simulink model "Simulate_position_motor_controllers"  (R2014b)
settings: Solver=ode23t  SolverMode=SingleTasking  StartTime=0.0  StopTime=simtime  RelTol=1e-3
values from neighbouring files (symbols this model uses):
  c0 = (s2 + s1 + s0)/(1 + r0)    [pbutest.m]    (also in workshop1.m)
  c0_ = (s2_ + s1_ + s0_)/(1 + r0)    [pbutest.m]    (also in workshop1.m)
  d0 = (r0*(s1 + s2) - s0)/(1 + r0)    [pbutest.m]    (also in workshop1.m)
  d0_ = (r0*(s1_ + s2_))/(1 + r0)    [pbutest.m]    (also in workshop1.m)
  d1 = s2    [pbutest.m]    (also in workshop1.m)
  d1_ = s2_    [pbutest.m]    (also in workshop1.m)
  F_c = 1.5e-3    (= 0.0015)    [continuous_design.m]    (also in workshop1.m)
  J1 = 0.0006    [continuous_design.m]    (also in workshop1.m)
  Kb = 10    [workshop1.m]
  motor = motor_pars    [continuous_design.m]    (also in workshop1.m)
  n = 5    [continuous_design.m]    (also in workshop1.m)
  r0 = 2*Zeta*omega3-b+omega1+omega2    [continuous_design.m]    (also in pbutest.m = (-b1^3*p1*p2*p3*p4-b0*b1^2*p1*p2*p3-b0*b1^2*p1*p2*p4-b0*b1^2; workshop1.m = (-b1^3*p1*p2*p3*p4-b0*b1^2*p1*p2*p3-b0*b1^2*p1*p2*p4-b0*b1^2)
  R_sim = Rd.num{1}    [pbutest.m]    (also in workshop1.m)
  S_sim = Sd.num{1}    [pbutest.m]    (also in workshop1.m)
  T_sim = Td.num{1}    [pbutest.m]    (also in workshop1.m)
  Ts = 2*pi/ws    [continuous_design.m]    (also in pbutest.m = 0.0108705628152; workshop1.m = 0.108705628152)
libraries: simulink x1
settings Model: Creator=Gabriel  LastModifiedBy=es2lab2
settings SolverCC: ZeroCrossAlgorithm=Adaptive
settings OptimizationCC: BlockReduction=off  BooleanDataType=off  UseDivisionForNetSlopeComputation=off  SimCompilerOptimization=off
settings DebuggingCC: SaveWithParameterizedLinksMsg=none  UnderspecifiedInitializationDetection=Classic  MergeDetectMultiDrivingBlocksExec=none  SignalResolutionControl=TryResolveAllWithWarning  SolverPrmCheckMsg=none  FrameProcessingCompatibilityMsg=error  AllowSymbolicDim=off
settings HardwareCC: TargetBitPerPointer=64  TargetLongLongMode=on  TargetIntDivRoundTo=Zero  TargetEndianess=LittleEndian  TargetWordSize=64  TargetHWDeviceType=MATLAB Host  ProdEqTarget=off
settings RTWCC: RTWCompilerOptimization=off
settings ConfigComp: CovMetricSettings=dw  CovHtmlReporting=on  CovSaveCumulativeToWorkspaceVar=on  CovSaveSingleToWorkspaceVar=on  CovModelRefEnable=Off  CovExternalEMLEnable=off  CovSFcnEnable=off

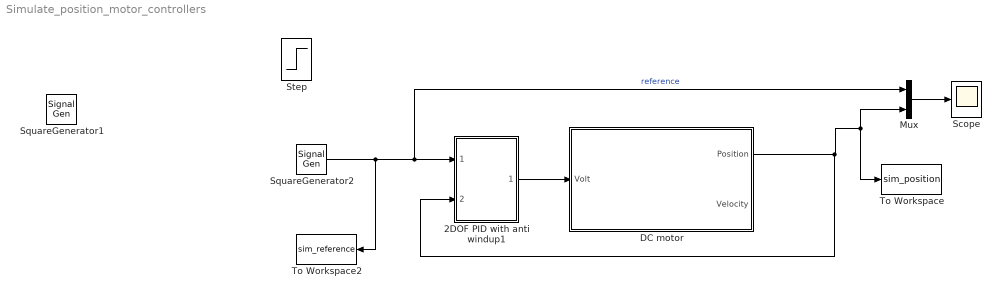
== system Simulate_position_motor_controllers ==
  2DOF PID with anti windup1 : Subsystem
  DC motor : Subsystem
  Mux : Mux  Inputs=2
  Scope : Scope
      settings: ShowLegends=on  TimeRange=7.551351351351352  YMin=-0.5  YMax=4.5
  SquareGenerator1 : SignalGenerator  WaveForm=square  Amplitude=4  Units=rad/sec
  SquareGenerator2 : SignalGenerator  WaveForm=square  Amplitude=4  Units=rad/sec
  Step : Step  Time=0  After=4  SampleTime=0
  To Workspace : ToWorkspace  VariableName=sim_position  SaveFormat=Timeseries  SampleTime=-1
  To Workspace2 : ToWorkspace  VariableName=sim_reference  SaveFormat=Timeseries  SampleTime=-1
  wires:
  SquareGenerator2/1 -> To Workspace2/1, Mux/1, 2DOF PID with anti windup1/1("reference ")  "reference"
  DC motor/1(Position) -> 2DOF PID with anti windup1/2(feedback), Mux/2, To Workspace/1
  2DOF PID with anti windup1/1(Voltage) -> DC motor/1(Volt)
  Mux/1 -> Scope/1

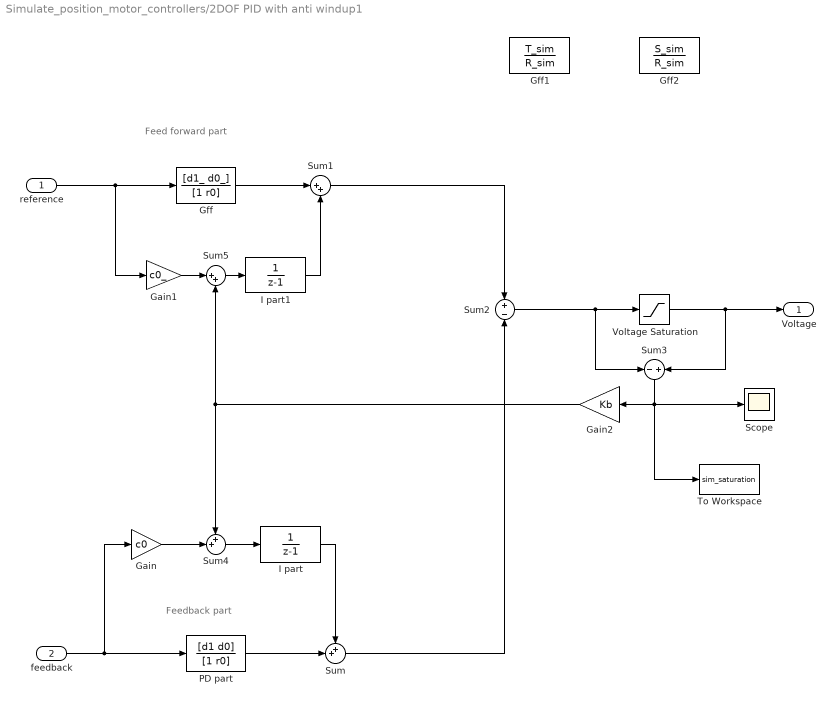
== system Simulate_position_motor_controllers/2DOF PID with anti windup1 ==
  note: Feedback part
  note: Feed forward part
  "reference " : Inport
  feedback : Inport  Port=2
  Gain : Gain  Gain=c0
  Gain1 : Gain  Gain=c0_
  Gain2 : Gain  Gain=Kb
  Gff : DiscreteTransferFcn  Numerator=[d1_ d0_]  Denominator=[1 r0]  SampleTime=Ts
  Gff1 : DiscreteTransferFcn  Numerator=T_sim  Denominator=R_sim  SampleTime=Ts
  Gff2 : DiscreteTransferFcn  Numerator=S_sim  Denominator=R_sim  SampleTime=Ts
  I part : DiscreteTransferFcn  Numerator=[0 1]  Denominator=[1 -1]  SampleTime=Ts
  I part1 : DiscreteTransferFcn  Numerator=[0 1]  Denominator=[1 -1]  SampleTime=Ts
  PD part : DiscreteTransferFcn  Numerator=[d1 d0]  Denominator=[1 r0]  SampleTime=Ts
  Scope : Scope
  Sum : Sum  Inputs=++|
  Sum1 : Sum  Inputs=|++
  Sum2 : Sum  Inputs=+|-
  Sum3 : Sum  Inputs=-|+
  Sum4 : Sum  Inputs=++|
  Sum5 : Sum  Inputs=|++
  To Workspace : ToWorkspace  VariableName=sim_saturation  SaveFormat=Timeseries  SampleTime=-1
  "Voltage Saturation " : Saturate  UpperLimit=24  LowerLimit=-24
  Voltage : Outport
  wires:
  "Voltage Saturation "/1 -> Sum3/2, Voltage/1
  "reference "/1 -> Gain1/1, Gff/1
  feedback/1 -> Gain/1, PD part/1
  Sum2/1 -> Sum3/1, "Voltage Saturation "/1
  Sum/1 -> Sum2/2
  Gff/1 -> Sum1/1
  I part1/1 -> Sum1/2
  Sum1/1 -> Sum2/1
  PD part/1 -> Sum/2
  I part/1 -> Sum/1
  Sum3/1 -> To Workspace/1, Scope/1, Gain2/1
  Sum4/1 -> I part/1
  Gain/1 -> Sum4/2
  Gain2/1 -> Sum5/2, Sum4/1
  Gain1/1 -> Sum5/1
  Sum5/1 -> I part1/1

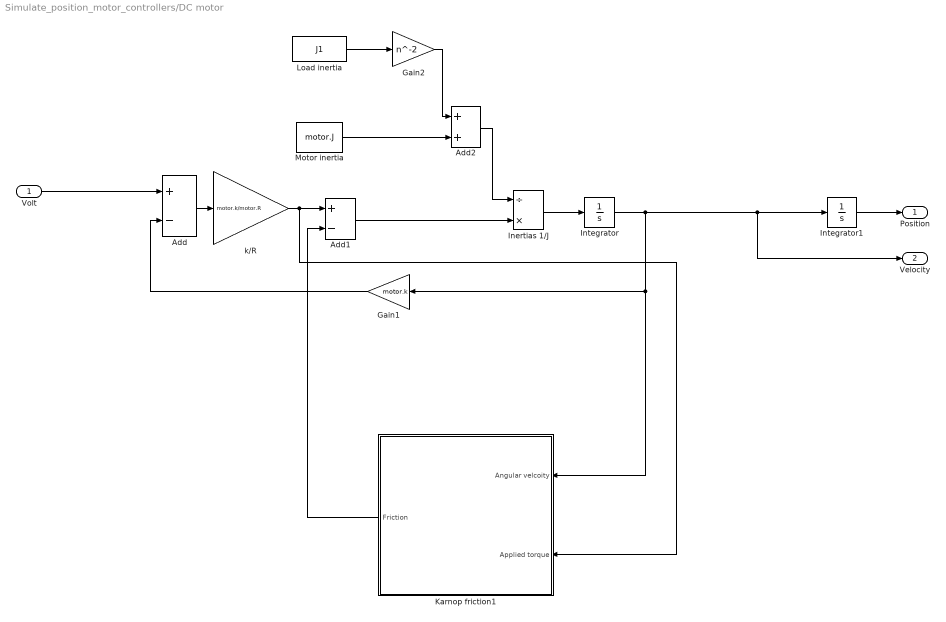
== system Simulate_position_motor_controllers/DC motor ==
  Volt : Inport
  Add : Sum  Inputs=+-
  Add1 : Sum  Inputs=+-
  Add2 : Sum
  Gain1 : Gain  Gain=motor.k
  Gain2 : Gain  Gain=n^-2
  Inertias 1/J : Product  Inputs=/*
  Integrator : Integrator
  Integrator1 : Integrator
  Karnop friction1 : Subsystem
  Load inertia : Constant  Value=J1
  Motor inertia : Constant  Value=motor.J
  "k/R " : Gain  Gain=motor.k/motor.R
  Position : Outport
  Velocity : Outport  Port=2
  wires:
  Karnop friction1/1(Friction) -> Add1/2
  Add2/1 -> Inertias 1/J/1
  Gain2/1 -> Add2/1
  Load inertia/1 -> Gain2/1
  Motor inertia/1 -> Add2/2
  Integrator/1 -> Integrator1/1, Velocity/1, Karnop friction1/1(Angular velcoity), Gain1/1
  Volt/1 -> Add/1
  Add1/1 -> Inertias 1/J/2
  Integrator1/1 -> Position/1
  Inertias 1/J/1 -> Integrator/1
  "k/R "/1 -> Add1/1, Karnop friction1/2(Applied torque)
  Add/1 -> "k/R "/1
  Gain1/1 -> Add/2

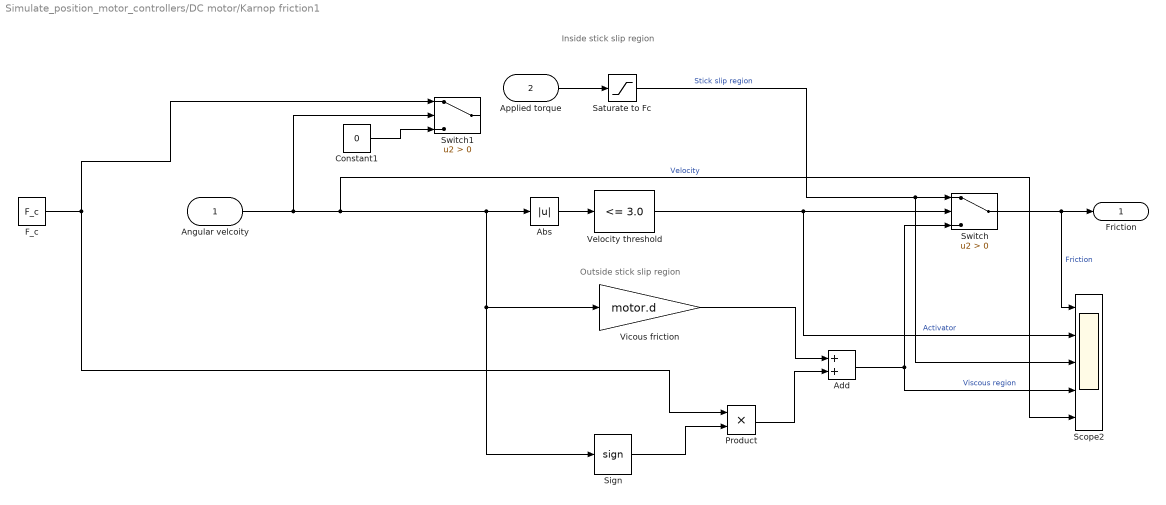
== system Simulate_position_motor_controllers/DC motor/Karnop friction1 ==
  note: Outside stick slip region
  note: Inside stick slip region
  Angular velcoity : Inport
  Applied torque : Inport  Port=2
  Abs : Abs  ZeroCross=off
  Add : Sum
  Constant1 : Constant  Value=0
  F_c : Constant  Value=F_c
  Product : Product
  Saturate to Fc : Saturate  UpperLimit=F_c  LowerLimit=-F_c  ZeroCross=off
  Scope2 : Scope  NumInputPorts=5
  Sign : Signum  ZeroCross=off
  Switch : Switch  Criteria=u2 > Threshold  ZeroCross=off
  Switch1 : Switch  Criteria=u2 > Threshold  ZeroCross=off
  "Velocity threshold " : simulink/Logic and Bit Operations/Compare To Constant  relop=<=  const=3.0  OutDataTypeStr=boolean
  Vicous friction : Gain  Gain=motor.d
  Friction : Outport
  wires:
  Applied torque/1 -> Saturate to Fc/1
  Add/1 -> Scope2/4, Switch/3  "Viscous region"
  Sign/1 -> Product/2
  F_c/1 -> Product/1, Switch1/1
  Vicous friction/1 -> Add/1
  Product/1 -> Add/2
  Abs/1 -> "Velocity threshold "/1
  "Velocity threshold "/1 -> Switch/2, Scope2/2  "Activator"
  Angular velcoity/1 -> Switch1/2, Sign/1, Vicous friction/1, Abs/1, Scope2/5  "Velocity"
  Switch/1 -> Friction/1, Scope2/1  "Friction"
  Saturate to Fc/1 -> Switch/1, Scope2/3  "Stick slip region"
  Constant1/1 -> Switch1/3
